simulink model "test_model"  (R2019b)
settings: Solver=VariableStepAuto  StartTime=0.0  StopTime=10.0  RelTol=1e-3
undefined symbols (not defined in the file): canChannel
libraries: canlib x3, canmsglib x2
settings Model: Creator=patri  LastModifiedBy=patri

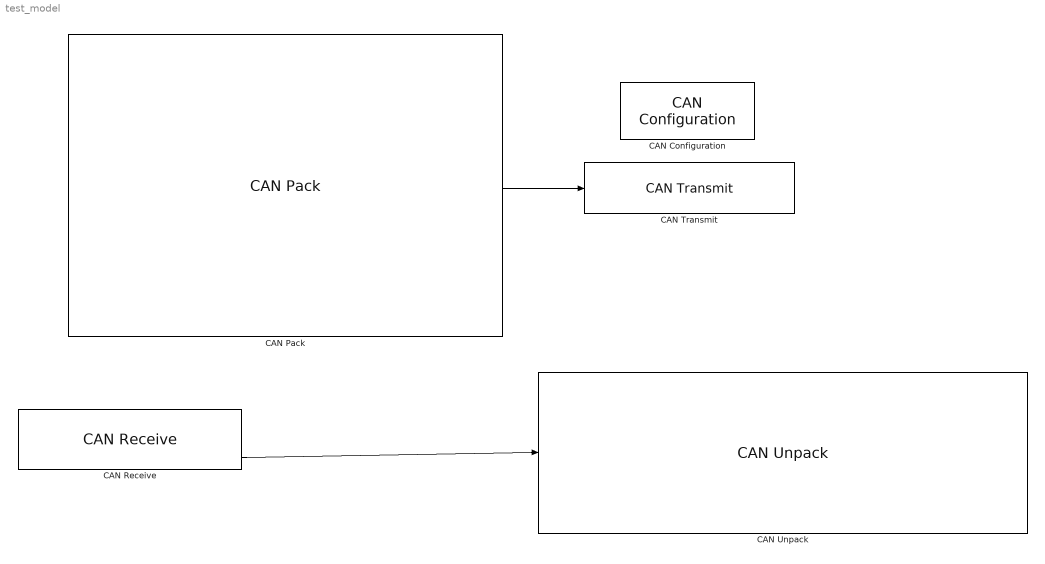
== system test_model ==
  CAN Configuration : canlib/CAN Configuration  BlockHandle=4.0001  Device=MathWorks Virtual 1 (Channel 1)  DeviceMenu=MathWorks Virtual 1 (Channel 1)  ObjConstructor=canChannel('MathWorks', 'Virtual 1', 1)  BusSpeed=500000  EnableBitParameters=off  AckMode=Normal
      settings: SourceProductName=Vehicle Network Toolbox  SourceProductBaseCode=VN
  CAN Pack : canmsglib/CAN Pack  CANdbFile=C:\Users\patri\OneDrive\Desktop\ts_20-code-development\CANBUS Database\ts_20-precharge_controller.dbc  MsgList=PRECHARGE_CONTROLLER_ERROR  MsgName=PRECHARGE_CONTROLLER_ERROR  MsgIDType=Standard (11-bit identifier)  MsgIdentifier=1089  MsgLength=4  Remote=off  ApplyMinMax=off  BusOutput=off  SignalInfo={'precharge_IMD_ok','8','1','LE','unsigned','Standard','0','1','0','-Inf','Inf';'precharge_PCB_overtemperature','24','1','LE','unsigned','Standard','0','1','0','-Inf','Inf';'precharge_PDOC_ok','9','1','LE','unsigned','Standard','0','1','0','-Inf','Inf';'precharge_cell_overtemperature','13','1','LE','unsigned','Standard','0','1','0','-Inf','Inf';'precharge_cell_overvoltage','12','1','LE','unsigned','Standard','0','1','0','-Inf','Inf';'precharge_cell_undervoltage','11','1','LE','unsigned','Standard','0','1','0','-Inf','Inf';'precharge_error_present','0','8','LE','unsigned','Standard','0','1','0','-Inf','Inf';'precharge_negative_AIR_mismatch','26','1','LE','unsigned','Standard','0','1','0','-Inf','Inf';'precharge_orion_disconnected','10','1','LE','unsigned','Standard','0','1','0','-Inf','Inf';'precharge_positive_AIR_mismatch','27','1','LE','unsigned','Standard','0','1','0','-Inf','Inf';'precharge_pre_dis_mismatch','25','1','LE','unsigned','Standard','0','1','0','-Inf','Inf';'precharge_warning_present','16','8','LE','unsigned','Standard','0','1','0','-Inf','Inf'}
      settings: SourceProductName=Vehicle Network Toolbox  SourceProductBaseCode=VN  DataFormat=CANdb specified signals
  CAN Receive : canlib/CAN Receive  BlockHandle=7.0001  Device=MathWorks Virtual 1 (Channel 1)  DeviceMenu=MathWorks Virtual 1 (Channel 1)  ObjConstructor=canChannel('MathWorks', 'Virtual 1', 1)  EnableStandardIDsFilter=off  StdIDsCombo=Allow all  StandardIDs=0  EnableExtendedIDsFilter=off  ExtIDsCombo=Allow all  ExtendedIDs=0  SampleTime=0.01  MsgsPerTimestep=all  InternalFilterUpdateStatus=on  BusOutput=off
      settings: SourceProductName=Vehicle Network Toolbox  SourceProductBaseCode=VN
  CAN Transmit : canlib/CAN Transmit  BlockHandle=9.0001  Device=MathWorks Virtual 1 (Channel 1)  DeviceMenu=MathWorks Virtual 1 (Channel 1)  ObjConstructor=canChannel('MathWorks', 'Virtual 1', 1)  EnablePeriodicTransmit=on  MessagePeriod=1.000
      settings: SourceProductName=Vehicle Network Toolbox  SourceProductBaseCode=VN
  CAN Unpack : canmsglib/CAN Unpack  CANdbFile=C:\Users\patri\OneDrive\Desktop\ts_20-code-development\CANBUS Database\ts_20-precharge_controller.dbc  MsgList=PRECHARGE_CONTROLLER_PERIPHERAL  MsgName=PRECHARGE_CONTROLLER_PERIPHERAL  MsgIDType=Standard (11-bit identifier)  MsgIdentifier=1091  MsgLength=6  SignalInfo={ 'precharge_AIR_neg_feedback', '40', '8', 'LE', 'unsigned', 'Standard', '0', '1', '0', '-Inf', 'Inf'; 'precharge_AIR_pos_feedback', '32', '8', 'LE', 'unsigned', 'Standard', '0', '1', '0', '-Inf', 'Inf'; 'precharge_AIR_power', '24', '8', 'LE', 'unsigned', 'Standard', '0', '1', '0', '-Inf', 'Inf'; 'precharge_IMD_duty_cycle', '16', '8', 'LE', 'unsigned', 'Standard', '0', '1', '0', '-Inf', 'Inf'; 'precharge_IMD_period', '8', '8', 'LE', 'unsigned', 'Standard', '0', '1', '0', '-Inf', 'Inf'; 'precharge_relay', '0', '8', 'LE', 'unsigned', 'Standard', '0', '1', '0', '-Inf', 'Inf' }  IDPort=off  TimestampPort=off  ErrorPort=off  RemotePort=off  LengthPort=off  StatusPort=off  ApplyMinMax=off
      settings: SourceProductName=Vehicle Network Toolbox  SourceProductBaseCode=VN  DataFormat=CANdb specified signals
  wires:
  CAN Pack/1 -> CAN Transmit/1
  CAN Receive/2 -> CAN Unpack/1
